simulink model "second_order_DE"  (R2020a)
settings: Solver=VariableStepAuto  StartTime=0.0  StopTime=10.0  RelTol=1e-3
settings Model: Creator=Riyansh  LastModifiedBy=Riyansh

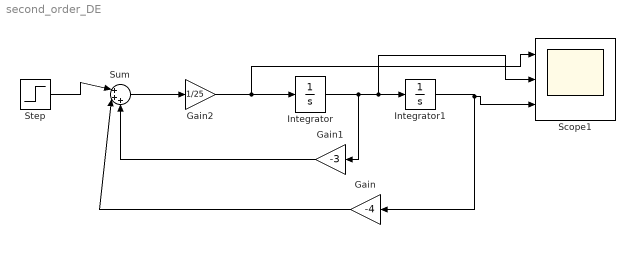
== system second_order_DE ==
  Gain : Gain  Gain=-4
  Gain1 : Gain  Gain=-3
  Gain2 : Gain  Gain=1/25
  Integrator : Integrator
  Integrator1 : Integrator
  Scope1 : Scope  NumInputPorts=3
  Step : Step  SampleTime=0
  Sum : Sum  Inputs=|+++
  wires:
  Integrator/1 -> Gain1/1, Scope1/2, Integrator1/1
  Integrator1/1 -> Scope1/3, Gain/1
  Step/1 -> Sum/1
  Gain1/1 -> Sum/3
  Gain/1 -> Sum/2
  Gain2/1 -> Scope1/1, Integrator/1
  Sum/1 -> Gain2/1
